simulink model "BMSTestHarness"  (R2024b)
settings: Solver=VariableStepAuto  StartTime=0.0  StopTime=20  RelTol=1e-3
PreLoadFcn:
  | BMSTestHarnessParams;
model workspace (MAT data in the model file):
  Cellvolt = Simulink.Parameter
  Cellvolt.Value = [1; 1; 1; 1; 1; 1; 1; 1; 1; 1]
  Cellvolt.Complexity = 'real'
  Cellvolt.Dimensions = [10 1]
  Cellvolt.DataType = 'auto'
  ModuleTemp = Simulink.Parameter
  ModuleTemp.Value = [1; 1; 1; 1; 1; 1; 1; 1; 1; 1]
  ModuleTemp.Complexity = 'real'
  ModuleTemp.Dimensions = [10 1]
  ModuleTemp.DataType = 'auto'
  ParVolt = Simulink.Parameter
  ParVolt.Value = [1; 1; 1; 1; 1; 1; 1; 1; 1; 1; 1; 1; 1; 1; 1; 1; 1; 1; 1; 1; 1; 1; 1; 1; 1; 1; 1; 1; 1; 1; 1; 1; 1; 1; 1; 1; 1; 1; 1; 1; 1; 1; 1; 1; 1; 1; 1; 1; 1; 1; 1; 1; 1; 1; 1; 1; 1; 1; 1; 1; 1; 1; 1; 1; 1; 1; 1; 1; 1; 1; 1; 1; 1; 1; 1; 1; 1; 1; 1; 1; 1; 1; 1; 1; 1; 1; 1; 1; 1; 1; 1; 1; 1; 1; 1; 1; 1; 1; 1; 1; 1; 1; 1; 1; 1; 1; 1; 1; 1; 1]
  ParVolt.Complexity = 'real'
  ParVolt.Dimensions = [110 1]
  ParVolt.DataType = 'auto'
  SoC = Simulink.Parameter
  SoC.Value = [1; 1; 1; 1; 1; 1; 1; 1; 1; 1]
  SoC.Complexity = 'real'
  SoC.Dimensions = [10 1]
  SoC.DataType = 'auto'
settings Model: Creator=jjha  LastModifiedBy=saprasad
settings OptimizationCC: ReuseModelBlockBuffer=off
settings RTWCC: GPUComputeCapability=3.5

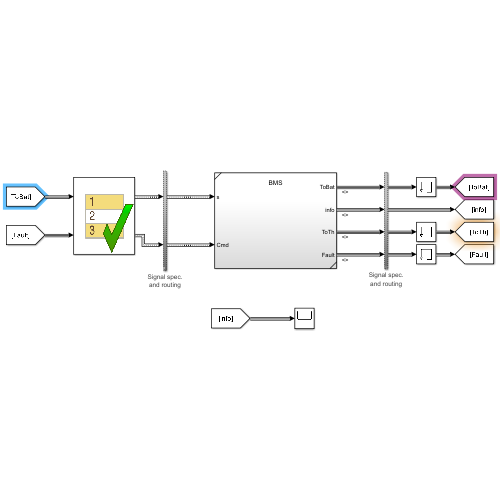
[thumbnail: Simulink's stored preview of the top-level diagram]
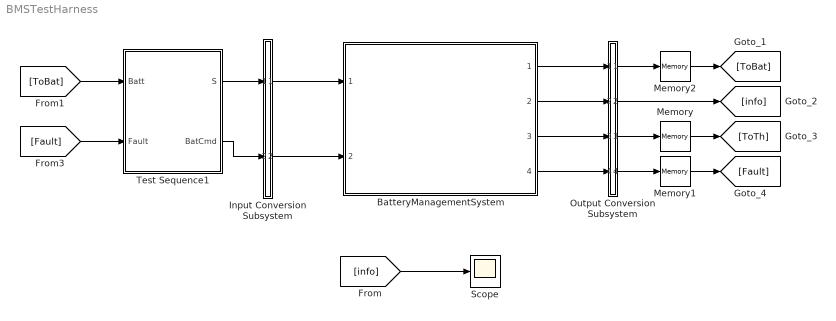
== system BMSTestHarness ==
  BatteryManagementSystem : Subsystem  ReferencedSubsystem=BMS
  Input Conversion Subsystem : Subsystem  Tag=__SLT_ICS__  Description=|
      | Signal spec.
      | and routing
      settings: AttributesFormatString=%<Description>
  Memory : Memory
  Memory1 : Memory
  Memory2 : Memory
  Output Conversion Subsystem : Subsystem  Tag=__SLT_OCS__  Description=|
      | Signal spec.
      | and routing
      settings: AttributesFormatString=%<Description>
  Scope : Scope
  Test Sequence1 : Test Sequence  TreatAsAtomicUnit=on
  wires:
  Test Sequence1/1(S) -> Input Conversion Subsystem/1(Inport_1)
  Test Sequence1/2(BatCmd) -> Input Conversion Subsystem/2(Inport_2)
  Input Conversion Subsystem/1(Outport_1) -> BatteryManagementSystem/1
  Input Conversion Subsystem/2(Outport_2) -> BatteryManagementSystem/2
  BatteryManagementSystem/1 -> Output Conversion Subsystem/1(Inport_1)
  BatteryManagementSystem/2 -> Output Conversion Subsystem/2(Inport_2)
  BatteryManagementSystem/3 -> Output Conversion Subsystem/3(Inport_3)
  BatteryManagementSystem/4 -> Output Conversion Subsystem/4(Inport_4)
  [Fault] -> Test Sequence1/2(Fault)
  [ToBat] -> Test Sequence1/1(Batt)
  Memory/1 -> [ToTh]
  Output Conversion Subsystem/3(Outport_3) -> Memory/1
  Memory2/1 -> [ToBat]
  Output Conversion Subsystem/2(Outport_2) -> [info]
  Output Conversion Subsystem/1(Outport_1) -> Memory2/1
  Output Conversion Subsystem/4(Outport_4) -> Memory1/1
  Memory1/1 -> [Fault]
  [info] -> Scope/1

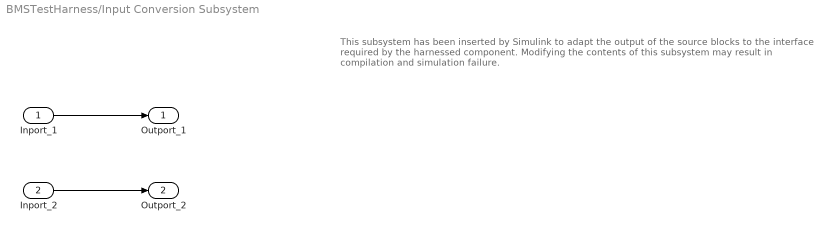
== system BMSTestHarness/Input Conversion Subsystem ==
  note: This subsystem has been inserted by Simulink to adapt the output of the source blocks to the interface required by the harnessed component.
      |  Modifying the contents of this subsystem may result in compilation and simulation failure.
  Inport_1 : Inport
  Inport_2 : Inport  Port=2
  Outport_1 : Outport
  Outport_2 : Outport  Port=2
  wires:
  Inport_1/1 -> Outport_1/1
  Inport_2/1 -> Outport_2/1

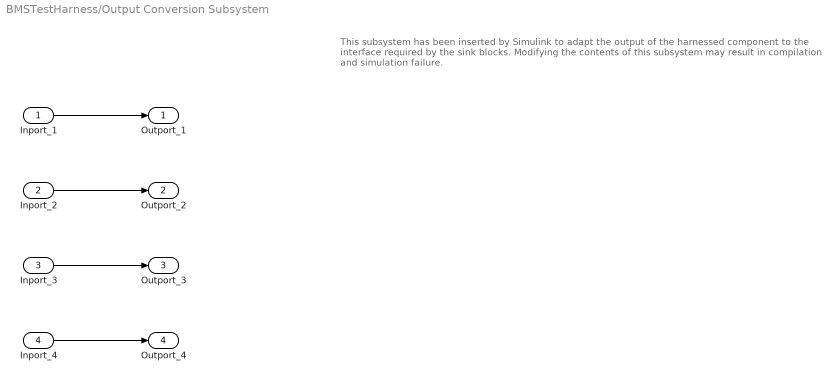
== system BMSTestHarness/Output Conversion Subsystem ==
  note: This subsystem has been inserted by Simulink to adapt the output of the harnessed component to the interface required by the sink blocks.
      |  Modifying the contents of this subsystem may result in compilation and simulation failure.
  Inport_1 : Inport
  Inport_2 : Inport  Port=2
  Inport_3 : Inport  Port=3
  Inport_4 : Inport  Port=4
  Outport_1 : Outport
  Outport_2 : Outport  Port=2
  Outport_3 : Outport  Port=3
  Outport_4 : Outport  Port=4
  wires:
  Inport_1/1 -> Outport_1/1
  Inport_2/1 -> Outport_2/1
  Inport_3/1 -> Outport_3/1
  Inport_4/1 -> Outport_4/1

== stateflow chart BMSTestHarness/Test Sequence1 ==
  state Scenario_1
    state Initialize_battery
      %% Initialize data outputs.
      S.temp = 295*ModuleTemp;
      S.ParVolt = 4*ParVolt;
      S.Cellvolt = 44*Cellvolt;
      S.Current = 0;
      S.SoC = .75*SoC;
      BatCmd.BatCmd=1;
      BatCmd.Reset=0;
    state Verify_batteryConnect
      verify(Batt.Relay.RelayPos >=1,'Battery Pos relay connected')
      verify(Batt.Relay.RelayNeg >=1,'Battery Pos relay connected')
      verify(abs(Batt.BatSt-1)<1E-6,'Battery status 1, in standby mode')
    state Battery_Discharge
      BatCmd.BatCmd=3;
    state Verify_batteryDischarging
      verify(Batt.Relay.RelayDchg >=1,'Battery Pos relay connected')
      verify(abs(Batt.BatSt-3)<1E-6,'Battery status 3, in discharge mode')
    state Battery_Charging
      BatCmd.BatCmd=2;
    state Verify_batteryCharging
      verify(Batt.Relay.RelayChg >=1,'Battery Pos relay connected')
      verify(abs(Batt.BatSt-2)<1E-6,'Battery status 2, in charge mode')
    state SoCmax_case
      S.SoC = .995*SoC;
    state Verify_SoCmaxOp
      verify(Batt.Relay.RelayChg <=0,'Battery Pos relay connected')
      verify(abs(Batt.BatSt-1)<1E-6,'Battery status 1,  in standby mode ')
    state SoCmaxDeactivate
      S.SoC = .85*SoC;
    state Verify_Charging
      verify(Batt.Relay.RelayChg >=1,'Battery Pos relay connected')
      verify(abs(Batt.BatSt-2)<1E-6,'Battery status 2, in charge mode')
    (default) -> Scenario_1.Initialize_battery
    Scenario_1.Initialize_battery -> Verify_batteryConnect : [
        | after(1,sec)
        | ]
    Verify_batteryConnect -> Battery_Discharge
    Battery_Discharge -> Verify_batteryDischarging : [
        | after(1,sec)
        | ]
    Verify_batteryDischarging -> Battery_Charging
    Battery_Charging -> Verify_batteryCharging : [
        | after(1,sec)
        | ]
    Verify_batteryCharging -> SoCmax_case
    SoCmax_case -> Verify_SoCmaxOp : [
        | after(1,sec)
        | ]
    Verify_SoCmaxOp -> SoCmaxDeactivate
    SoCmaxDeactivate -> Verify_Charging : [
        | after(1,sec)
        | ]
  state Scenario_2
    state Initialize_battery
      %% Initialize data outputs.
      S.temp = 295*ModuleTemp;
      S.ParVolt = 4*ParVolt;
      S.Cellvolt = 44*Cellvolt;
      S.Current = 0;
      S.SoC = .75*SoC;
      BatCmd.BatCmd=1;
      BatCmd.Reset=0;
      state DischargeMode_activate
        BatCmd.BatCmd=3;
      state Discharging_active
        S.Current = -30;
      state else
      Scenario_2.Initialize_battery -> (junction 196) [order 1]
      (default) -> (junction 196)
      (junction 196) -> (junction 197) [order 1] : [Batt.BatSt==1
          | ]
      (junction 197) -> DischargeMode_activate [order 1] : [~in(Scenario_2.Initialize_battery.DischargeMode_activate)]
      (junction 196) -> (junction 204) [order 2]
      (junction 197) -> (junction 200) [order 2]
      (junction 204) -> (junction 205) [order 1] : [Batt.BatSt==3
          | ]
      (junction 205) -> Discharging_active [order 1] : [~in(Scenario_2.Initialize_battery.Discharging_active)]
      (junction 205) -> (junction 208) [order 2]
      (junction 221) -> (junction 222)
      (junction 222) -> else [order 1] : [~in(Scenario_2.Initialize_battery.else)]
      (junction 222) -> (junction 225) [order 2]
      (junction 204) -> (junction 221) [order 2]
    state DischargeFault_activate
      S.Current=-700
    state DischargeFault_active
      verify(abs(Fault.Fault.FaultElec.Dchg -1)<1E-6,'Discharge Fault triggered')
    (default) -> Scenario_2.Initialize_battery
    Scenario_2.Initialize_battery -> DischargeFault_activate [order 1]
    DischargeFault_activate -> DischargeFault_active : [
        | after(5,sec)
        | ]
  (default) -> Scenario_1 [order 1] : [Active_Scenario_Index == 1]
  (default) -> Scenario_2 [order 2] : {assert(Active_Scenario_Index == 2,'The value of Scenario Parameter ''Active_Scenario_Index'' is not valid. Use the index of the scenario to specify it.')}
  data: S output Bus: Sensor size=1; Batt input Bus: Batt; Fault input Bus: FaultBus; ModuleTemp parameter; ParVolt parameter; Cellvolt parameter; SoC parameter; BatCmd output Bus: BatCmd; Active_Scenario_Index parameter =1
